simulink model "PID_Arduino3"  (R2024b)
settings: Solver=FixedStepAuto  StartTime=0.0  StopTime=30  RelTol=1e-3  EnableMultiTasking=on
values from neighbouring files (symbols this model uses):
  Kp_PI_tyr = Ku / 3.2    (= 9.6875)    [parameters.m]
  Kp_PID_zig = 0.6 * Ku    (= 18.6)    [parameters.m]
  Td_PID_zig = Pu / 8    (= 0.013125)    [parameters.m]
  Ti_PI_tyr = 2.2 * Pu    (= 0.231)    [parameters.m]
  Ti_PID_zig = Pu / 2    (= 0.0525)    [parameters.m]
libraries: arduinolib x10, slpidlib x2
settings Model: SimulationMode=external  ExtModeTrigDuration=2  Creator=bodro  LastModifiedBy=bodro
settings SolverCC: AutoInsertRateTranBlk=on
settings OptimizationCC: EnhancedBackFolding=on  PassReuseOutputArgsAs=Individual arguments  ZeroExternalMemoryAtStartup=off  ZeroInternalMemoryAtStartup=off  MaxStackSize=64  OptimizeBlockOrder=speed  DifferentSizesBufferReuse=on  OptimizationCustomize=off  EfficientTunableParamExpr=on
settings DebuggingCC: ParameterTunabilityLossMsg=error
settings HardwareCC: ProdBitPerPointer=32  ProdBitPerSizeT=32  ProdBitPerPtrDiffT=32  ProdLargestAtomicInteger=Long  ProdLargestAtomicFloat=Double  ProdWordSize=32  ProdHWDeviceType=ARM Compatible->ARM Cortex  UseEmbeddedCoderFeatures=off
settings SFSimCC: MATLABDynamicMemAlloc=off
settings RTWCC: Description=Embedded Coder  SystemTargetFile=ert.tlc  HardwareBoard=Arduino Due  TemplateMakefile=ert_default_tmf  Toolchain=Arduino ARM  BuildConfiguration=Faster Runs
settings CodeAppCC: ForceParamTrailComments=on  IgnoreCustomStorageClasses=off  OperatorAnnotations=on  SimulinkDataObjDesc=on  SFDataObjDesc=on  InsertBlockDesc=on
settings ERTTargetCC: SupportContinuousTime=on  SupportNonInlinedSFcns=on  SupportVariableSizeSignals=on  ExtModeTransport=3  ExtModeStaticAlloc=on  ExtModeAutomaticAllocSize=off  ExtModeStaticAllocSize=24576  ExtModeMexFile=ext_xcp  ExtModeIntrfLevel=Level2 - Open  InlinedParameterPlacement=Hierarchical

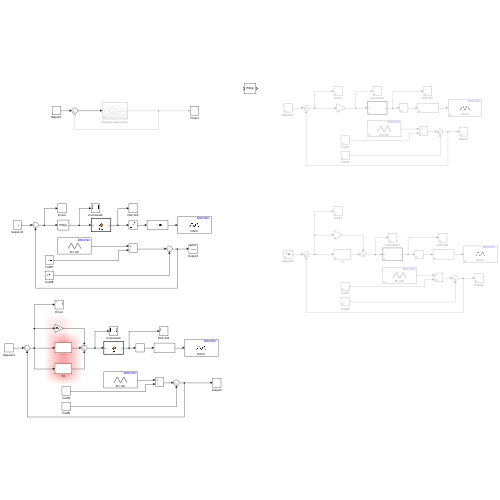
[thumbnail: Simulink's stored preview of the top-level diagram]
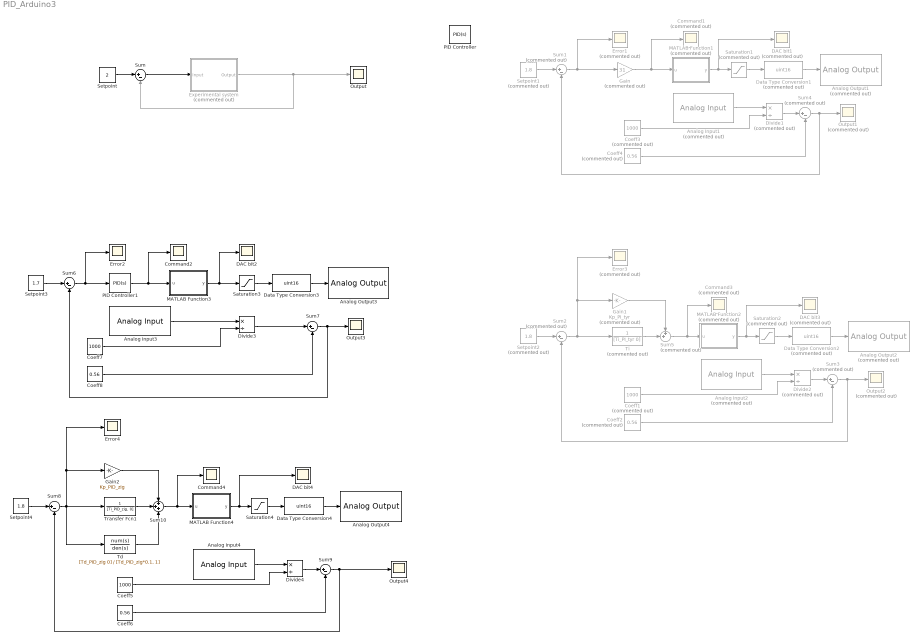
== system PID_Arduino3 ==
  Analog Input1 : arduinolib/Analog Input  Commented=on  pinNumber=8  ReadResultsOnly=off  ConversionTriggerSource=Software  ExternalTriggerType=uint32( 0 )  OutputDataType=uint16  EnableConversionCompleteNotify=off  EnableOuputStatus=off  SampleTime=0.001  blockPlatform=arduino
  Analog Input2 : arduinolib/Analog Input  Commented=on  pinNumber=8  ReadResultsOnly=off  ConversionTriggerSource=Software  ExternalTriggerType=uint32( 0 )  OutputDataType=uint16  EnableConversionCompleteNotify=off  EnableOuputStatus=off  SampleTime=0.001  blockPlatform=arduino
  Analog Input3 : arduinolib/Analog Input  pinNumber=8  ReadResultsOnly=off  ConversionTriggerSource=Software  ExternalTriggerType=uint32( 0 )  OutputDataType=uint16  EnableConversionCompleteNotify=off  EnableOuputStatus=off  SampleTime=0.001  blockPlatform=arduino
  Analog Input4 : arduinolib/Analog Input  pinNumber=8  ReadResultsOnly=off  ConversionTriggerSource=Software  ExternalTriggerType=uint32( 0 )  OutputDataType=uint16  EnableConversionCompleteNotify=off  EnableOuputStatus=off  SampleTime=0.001  blockPlatform=arduino
  Analog Output1 : arduinolib/Analog Output  Commented=on  blockPlatform=ARDUINO  DACpin=DAC0
  Analog Output2 : arduinolib/Analog Output  Commented=on  blockPlatform=ARDUINO  DACpin=DAC0
  Analog Output3 : arduinolib/Analog Output  blockPlatform=ARDUINO  DACpin=DAC0
  Analog Output4 : arduinolib/Analog Output  blockPlatform=ARDUINO  DACpin=DAC0
  Coeff1 : Constant  Commented=on  Value=1000
  Coeff2 : Constant  Commented=on  Value=0.56
  Coeff3 : Constant  Commented=on  Value=1000
  Coeff4 : Constant  Commented=on  Value=0.56
  Coeff5 : Constant  Value=1000
  Coeff6 : Constant  Value=0.56
  Coeff7 : Constant  Value=1000
  Coeff8 : Constant  Value=0.56
  Command1 : Scope  Commented=on
  Command2 : Scope
  Command3 : Scope  Commented=on
  Command4 : Scope
  DAC bit1 : Scope  Commented=on
  DAC bit2 : Scope
  DAC bit3 : Scope  Commented=on
  DAC bit4 : Scope
  Data Type Conversion1 : DataTypeConversion  Commented=on  OutDataTypeStr=uint16  SaturateOnIntegerOverflow=off  RndMeth=Floor
  Data Type Conversion2 : DataTypeConversion  Commented=on  OutDataTypeStr=uint16  SaturateOnIntegerOverflow=off  RndMeth=Floor
  Data Type Conversion3 : DataTypeConversion  OutDataTypeStr=uint16  SaturateOnIntegerOverflow=off  RndMeth=Floor
  Data Type Conversion4 : DataTypeConversion  OutDataTypeStr=uint16  SaturateOnIntegerOverflow=off  RndMeth=Floor
  Divide1 : Product  Commented=on  Inputs=*/
  Divide2 : Product  Commented=on  Inputs=*/
  Divide3 : Product  Inputs=*/
  Divide4 : Product  Inputs=*/
  Error1 : Scope  Commented=on
  Error2 : Scope
  Error3 : Scope  Commented=on
  Error4 : Scope
  Experimental system : Subsystem  Commented=on
  Gain : Gain  Commented=on  Gain=31
  Gain1 : Gain  Commented=on  Gain=Kp_PI_tyr
  Gain2 : Gain  Gain=Kp_PID_zig
  MATLAB Function1 : MATLAB Function  Commented=on  TreatAsAtomicUnit=on
  MATLAB Function2 : MATLAB Function  Commented=on  TreatAsAtomicUnit=on
  MATLAB Function3 : MATLAB Function  TreatAsAtomicUnit=on
  MATLAB Function4 : MATLAB Function  TreatAsAtomicUnit=on
  Output : Scope
  Output1 : Scope  Commented=on
  Output2 : Scope  Commented=on
  Output3 : Scope
  Output4 : Scope
  PID Controller : slpidlib/PID Controller  Controller=PID  Form=Parallel  TimeDomain=Continuous-time  UseExternalTs=off  SampleTime=-1  IntegratorMethod=Forward Euler  FilterMethod=Forward Euler  ControllerParametersSource=internal  P=15.01  I=230  UseKiTs=off  D=0.24  UseExternalDerivativeSource=off  N=100  UseFilter=on  TunerSelectOption=Transfer Function Based (PID Tuner App)  InitialConditionSource=internal  InitialConditionForIntegrator=0  InitialConditionForFilter=0  DifferentiatorICPrevScaledInput=0  ExternalReset=none  TrackingMode=off  Kt=1  LimitOutput=off  SatLimitsSource=internal  UpperSaturationLimit=inf  LowerSaturationLimit=-inf  LinearizeAsGain=on  AntiWindupMode=none  Kb=1  LimitIntegrator=off  UpperIntegratorSaturationLimit=inf  LowerIntegratorSaturationLimit=-inf  POutMin=[]  POutMax=[]  IOutMin=[]  IOutMax=[]  DOutMin=[]  DOutMax=[]  NOutMin=[]  NOutMax=[]  SumOutMin=[]  SumOutMax=[]  SaturationOutMin=[]  SaturationOutMax=[]  PParamMin=[]  PParamMax=[]  IParamMin=[]  IParamMax=[]  DParamMin=[]  DParamMax=[]  NParamMin=[]  NParamMax=[]  KbParamMin=[]  KbParamMax=[]  KtParamMin=[]  KtParamMax=[]  KbOutMin=[]  KbOutMax=[]  KtOutMin=[]  KtOutMax=[]  IntegratorOutMin=[]  IntegratorOutMax=[]  FilterOutMin=[]  FilterOutMax=[]  SumI1OutMin=[]  SumI1OutMax=[]  SumI2OutMin=[]  SumI2OutMax=[]  SumI3OutMin=[]  SumI3OutMax=[]  SumI4OutMin=[]  SumI4OutMax=[]  SumDOutMin=[]  SumDOutMax=[]  DifferentiatorOutMin=[]  DifferentiatorOutMax=[]  FilterDiffOutCoefMin=[]  FilterDiffOutCoefMax=[]  ReciprocalOutMin=[]  ReciprocalOutMax=[]  SumDenOutMin=[]  SumDenOutMax=[]  SumNumOutMin=[]  SumNumOutMax=[]  DivideOutMin=[]  DivideOutMax=[]  UdiffTsProdOutMin=[]  UdiffTsProdOutMax=[]  NTsProdOutMin=[]  NTsProdOutMax=[]  UintegralTsProdOutMin=[]  UintegralTsProdOutMax=[]  UngainTsProdOutMin=[]  UngainTsProdOutMax=[]  ClampingZeroOutDataTypeStr=Inherit: Inherit via back propagation  ClampingZeroOutMin=[]  ClampingZeroOutMax=[]  FilterDenConstantOutDataTypeStr=Inherit: Inherit via back propagation  FilterDenConstantOutMin=[]  FilterDenConstantOutMax=[]  PCopyOutDataTypeStr=Inherit: Inherit via back propagation  PCopyOutMin=[]  PCopyOutMax=[]  NCopyOutDataTypeStr=Inherit: Inherit via back propagation  NCopyOutMin=[]  NCopyOutMax=[]  IntegratorContinuousStateAttributes=''  IntegratorStateMustResolveToSignalObject=off  IntegratorRTWStateStorageClass=Auto  FilterContinuousStateAttributes=''  FilterStateMustResolveToSignalObject=off  FilterRTWStateStorageClass=Auto  ParallelPVariant=InternalParameters  IdealPVariant=Disabled  IVariant=InternalParameters  DVariant=InternalParameters  IntegratorVariant=Continuous  SatVariant=Disabled  AWVariant=Passthrough  PCopyVariant=Disabled  TRVariant=Disabled  FdbkBlocksVariant=Forward  IdealPFdbkVariant=Disabled  SatFdbkVariant=Disabled  DerivativeFilterVariant=ContFilter  NVariant=InternalParameters  NCopyVariant=Disabled  FilterICVariant=InternalICsFilter  IntegratorICVariant=InternalICs  ExternalResetVariant=Disabled  TRSumVariant=Passthrough  SumFdbkVariant=Disabled  SumVariant=Sum_PID  TsampFilterVariant=InternalTs  TsampNgainVariant=Passthrough  TsampIntegralVariant=Disabled_SignalSpec  ExternalSaturationOutDataTypeStr=Inherit: Same as second input  DerivativeSourceVariant=ErrorSignal  PreIntVariant=InternalPreInt
  PID Controller1 : slpidlib/PID Controller  Controller=PID  Form=Parallel  TimeDomain=Continuous-time  UseExternalTs=off  SampleTime=-1  IntegratorMethod=Forward Euler  FilterMethod=Forward Euler  ControllerParametersSource=internal  P=15.01  I=0.065  UseKiTs=off  D=0.016  UseExternalDerivativeSource=off  N=10  UseFilter=on  TunerSelectOption=Transfer Function Based (PID Tuner App)  InitialConditionSource=internal  InitialConditionForIntegrator=0  InitialConditionForFilter=0  DifferentiatorICPrevScaledInput=0  ExternalReset=none  TrackingMode=off  Kt=1  LimitOutput=off  SatLimitsSource=internal  UpperSaturationLimit=inf  LowerSaturationLimit=-inf  LinearizeAsGain=on  AntiWindupMode=none  Kb=1  LimitIntegrator=off  UpperIntegratorSaturationLimit=inf  LowerIntegratorSaturationLimit=-inf  POutMin=[]  POutMax=[]  IOutMin=[]  IOutMax=[]  DOutMin=[]  DOutMax=[]  NOutMin=[]  NOutMax=[]  SumOutMin=[]  SumOutMax=[]  SaturationOutMin=[]  SaturationOutMax=[]  PParamMin=[]  PParamMax=[]  IParamMin=[]  IParamMax=[]  DParamMin=[]  DParamMax=[]  NParamMin=[]  NParamMax=[]  KbParamMin=[]  KbParamMax=[]  KtParamMin=[]  KtParamMax=[]  KbOutMin=[]  KbOutMax=[]  KtOutMin=[]  KtOutMax=[]  IntegratorOutMin=[]  IntegratorOutMax=[]  FilterOutMin=[]  FilterOutMax=[]  SumI1OutMin=[]  SumI1OutMax=[]  SumI2OutMin=[]  SumI2OutMax=[]  SumI3OutMin=[]  SumI3OutMax=[]  SumI4OutMin=[]  SumI4OutMax=[]  SumDOutMin=[]  SumDOutMax=[]  DifferentiatorOutMin=[]  DifferentiatorOutMax=[]  FilterDiffOutCoefMin=[]  FilterDiffOutCoefMax=[]  ReciprocalOutMin=[]  ReciprocalOutMax=[]  SumDenOutMin=[]  SumDenOutMax=[]  SumNumOutMin=[]  SumNumOutMax=[]  DivideOutMin=[]  DivideOutMax=[]  UdiffTsProdOutMin=[]  UdiffTsProdOutMax=[]  NTsProdOutMin=[]  NTsProdOutMax=[]  UintegralTsProdOutMin=[]  UintegralTsProdOutMax=[]  UngainTsProdOutMin=[]  UngainTsProdOutMax=[]  ClampingZeroOutDataTypeStr=Inherit: Inherit via back propagation  ClampingZeroOutMin=[]  ClampingZeroOutMax=[]  FilterDenConstantOutDataTypeStr=Inherit: Inherit via back propagation  FilterDenConstantOutMin=[]  FilterDenConstantOutMax=[]  PCopyOutDataTypeStr=Inherit: Inherit via back propagation  PCopyOutMin=[]  PCopyOutMax=[]  NCopyOutDataTypeStr=Inherit: Inherit via back propagation  NCopyOutMin=[]  NCopyOutMax=[]  IntegratorContinuousStateAttributes=''  IntegratorStateMustResolveToSignalObject=off  IntegratorRTWStateStorageClass=Auto  FilterContinuousStateAttributes=''  FilterStateMustResolveToSignalObject=off  FilterRTWStateStorageClass=Auto  ParallelPVariant=InternalParameters  IdealPVariant=Disabled  IVariant=InternalParameters  DVariant=InternalParameters  IntegratorVariant=Continuous  SatVariant=Disabled  AWVariant=Passthrough  PCopyVariant=Disabled  TRVariant=Disabled  FdbkBlocksVariant=Forward  IdealPFdbkVariant=Disabled  SatFdbkVariant=Disabled  DerivativeFilterVariant=ContFilter  NVariant=InternalParameters  NCopyVariant=Disabled  FilterICVariant=InternalICsFilter  IntegratorICVariant=InternalICs  ExternalResetVariant=Disabled  TRSumVariant=Passthrough  SumFdbkVariant=Disabled  SumVariant=Sum_PID  TsampFilterVariant=InternalTs  TsampNgainVariant=Passthrough  TsampIntegralVariant=Disabled_SignalSpec  ExternalSaturationOutDataTypeStr=Inherit: Same as second input  DerivativeSourceVariant=ErrorSignal  PreIntVariant=InternalPreInt
  Saturation1 : Saturate  Commented=on  UpperLimit=4094  LowerLimit=1
  Saturation2 : Saturate  Commented=on  UpperLimit=4094  LowerLimit=1
  Saturation3 : Saturate  UpperLimit=4094  LowerLimit=1
  Saturation4 : Saturate  UpperLimit=4094  LowerLimit=1
  Setpoint : Constant  Value=2
  Setpoint1 : Constant  Commented=on  Value=1.8
  Setpoint2 : Constant  Commented=on  Value=1.8
  Setpoint3 : Constant  Value=1.7
  Setpoint4 : Constant  Value=1.8
  Sum{,6..9} (5 alike) : Sum  Inputs=|+-
  Sum{1..4} (4 alike) : Sum  Commented=on  Inputs=|+-
  Sum10 : Sum  Inputs=+++
  Sum5 : Sum  Commented=on  Inputs=++|
  Td : TransferFcn  Numerator=[Td_PID_zig 0]  Denominator=[Td_PID_zig*0.1, 1]
  Ti : TransferFcn  Commented=on  Denominator=[Ti_PI_tyr 0]
  Transfer Fcn1 : TransferFcn  Denominator=[Ti_PID_zig, 0]
  wires:
  Setpoint1/1 -> Sum1/1
  Sum1/1 -> Gain/1, Error1/1
  MATLAB Function1/1(y) -> DAC bit1/1, Saturation1/1
  Divide1/1 -> Sum4/1
  Analog Input1/1 -> Divide1/1
  Saturation1/1 -> Data Type Conversion1/1
  Sum4/1 -> Output1/1, Sum1/2
  Coeff3/1 -> Divide1/2
  Coeff4/1 -> Sum4/2
  Setpoint/1 -> Sum/1
  Data Type Conversion1/1 -> Analog Output1/1
  Data Type Conversion3/1 -> Analog Output3/1
  PID Controller1/1 -> MATLAB Function3/1(u), Command2/1
  Coeff8/1 -> Sum7/2
  Saturation3/1 -> Data Type Conversion3/1
  Coeff7/1 -> Divide3/2
  Divide3/1 -> Sum7/1
  Analog Input3/1 -> Divide3/1
  Setpoint3/1 -> Sum6/1
  MATLAB Function3/1(y) -> Saturation3/1, DAC bit2/1
  Sum6/1 -> PID Controller1/1, Error2/1
  Sum7/1 -> Output3/1, Sum6/2
  Sum/1 -> Experimental system/1(Input)
  Experimental system/1(Output) -> Output/1, Sum/2
  Gain/1 -> Command1/1, MATLAB Function1/1(u)
  Data Type Conversion2/1 -> Analog Output2/1
  MATLAB Function2/1(y) -> DAC bit3/1, Saturation2/1
  Coeff2/1 -> Sum3/2
  Saturation2/1 -> Data Type Conversion2/1
  Coeff1/1 -> Divide2/2
  Sum2/1 -> Ti/1, Gain1/1, Error3/1
  Sum3/1 -> Output2/1, Sum2/2
  Analog Input2/1 -> Divide2/1
  Divide2/1 -> Sum3/1
  Setpoint2/1 -> Sum2/1
  Sum5/1 -> Command3/1, MATLAB Function2/1(u)
  Gain1/1 -> Sum5/1
  Ti/1 -> Sum5/2
  Gain2/1 -> Sum10/1
  Setpoint4/1 -> Sum8/1
  Divide4/1 -> Sum9/1
  Analog Input4/1 -> Divide4/1
  Sum9/1 -> Output4/1, Sum8/2
  Transfer Fcn1/1 -> Sum10/2
  Data Type Conversion4/1 -> Analog Output4/1
  Saturation4/1 -> Data Type Conversion4/1
  MATLAB Function4/1(y) -> DAC bit4/1, Saturation4/1
  Coeff5/1 -> Divide4/2
  Coeff6/1 -> Sum9/2
  Td/1 -> Sum10/3
  Sum8/1 -> Td/1, Error4/1, Gain2/1, Transfer Fcn1/1
  Sum10/1 -> MATLAB Function4/1(u), Command4/1

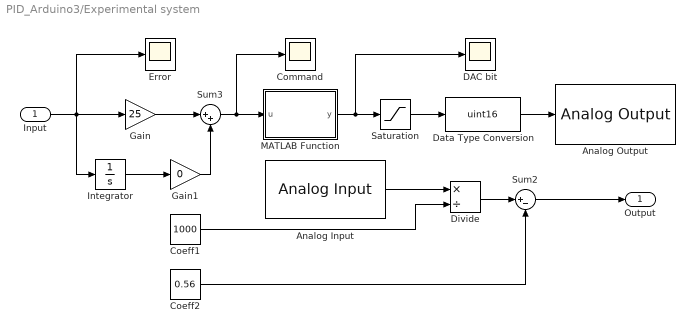
== system PID_Arduino3/Experimental system ==
  Input : Inport
  Analog Input : arduinolib/Analog Input  pinNumber=8  ReadResultsOnly=off  ConversionTriggerSource=Software  ExternalTriggerType=uint32( 0 )  OutputDataType=uint16  EnableConversionCompleteNotify=off  EnableOuputStatus=off  SampleTime=0.001  blockPlatform=arduino
  Analog Output : arduinolib/Analog Output  blockPlatform=ARDUINO  DACpin=DAC0
  Coeff1 : Constant  Value=1000
  Coeff2 : Constant  Value=0.56
  Command : Scope
  DAC bit : Scope
  Data Type Conversion : DataTypeConversion  OutDataTypeStr=uint16  SaturateOnIntegerOverflow=off  RndMeth=Floor
  Divide : Product  Inputs=*/
  Error : Scope
  Gain : Gain  Gain=25
  Gain1 : Gain  Gain=0
  Integrator : Integrator
  MATLAB Function : MATLAB Function  TreatAsAtomicUnit=on
  Saturation : Saturate  UpperLimit=4094  LowerLimit=1
  Sum2 : Sum  Inputs=|+-
  Sum3 : Sum  Inputs=|++
  Output : Outport
  wires:
  MATLAB Function/1(y) -> DAC bit/1, Saturation/1
  Gain/1 -> Sum3/1
  Divide/1 -> Sum2/1
  Analog Input/1 -> Divide/1
  Integrator/1 -> Gain1/1
  Input/1 -> Error/1, Integrator/1, Gain/1
  Sum3/1 -> MATLAB Function/1(u), Command/1
  Coeff1/1 -> Divide/2
  Data Type Conversion/1 -> Analog Output/1
  Saturation/1 -> Data Type Conversion/1
  Coeff2/1 -> Sum2/2
  Gain1/1 -> Sum3/2
  Sum2/1 -> Output/1

== matlab function PID_Arduino3/Experimental system/MATLAB Function ==
  data: u input; y output
function y = fcn(u)

V_offset = 0.56;
V_ref = 2.2;
N = 12;


y = ((2^N-1)/V_ref)*(u - V_offset);

== matlab function PID_Arduino3/MATLAB Function2 ==
  data: u input; y output
function y = fcn(u)

V_offset = 0.56;
V_ref = 2.2;
N = 12;


y = ((2^N-1)/V_ref)*(u - V_offset);

== matlab function PID_Arduino3/MATLAB Function3 ==
  data: u input; y output
function y = fcn(u)

V_offset = 0.56;
V_ref = 2.2;
N = 12;


y = ((2^N-1)/V_ref)*(u - V_offset);

== matlab function PID_Arduino3/MATLAB Function4 ==
  data: u input; y output
function y = fcn(u)

V_offset = 0.56;
V_ref = 2.2;
N = 12;


y = ((2^N-1)/V_ref)*(u - V_offset);

== matlab function PID_Arduino3/MATLAB Function1 ==
  data: u input; y output
function y = fcn(u)

V_offset = 0.56;
V_ref = 2.2;
N = 12;


y = ((2^N-1)/V_ref)*(u - V_offset);
